simulink model "Lipschtiz_solution"  (R2024b)
settings: Solver=VariableStepAuto  StartTime=0.0  StopTime=10.0  RelTol=1e-3
settings Model: Creator=david  LastModifiedBy=david

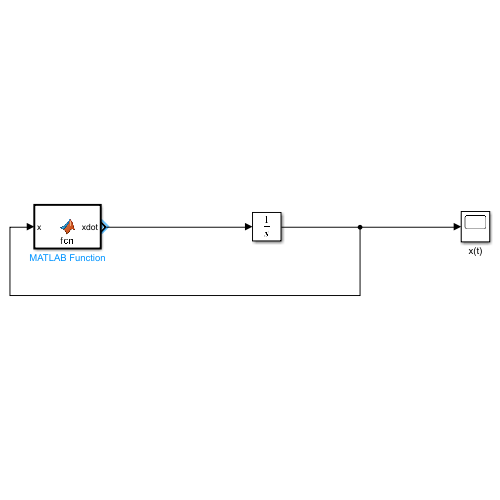
[thumbnail: Simulink's stored preview of the top-level diagram]
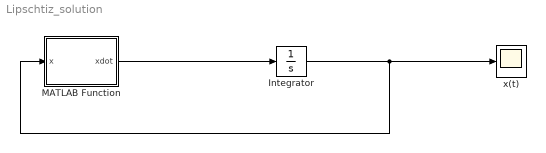
== system Lipschtiz_solution ==
  Integrator : Integrator  InitialCondition=1
  MATLAB Function : MATLAB Function  TreatAsAtomicUnit=on
  x(t) : Scope
  wires:
  Integrator/1 -> MATLAB Function/1(x), x(t)/1
  MATLAB Function/1(xdot) -> Integrator/1

== matlab function Lipschtiz_solution/MATLAB Function ==
  data: x input; xdot output
function xdot = fcn(x)

xdot = x^2;
